simulink model "MassSpringDamper"  (R2015b)
settings: Solver=VariableStepAuto  StartTime=0.0  StopTime=10  RelTol=1e-3
values from neighbouring files (symbols this model uses):
  b = 2    [MassDamperSpring.m]
  F = 1    [MassDamperSpring.m]
  k = 20    [MassDamperSpring.m]
  m = 1    [MassDamperSpring.m]
settings Model: Creator=DCLAP  LastModifiedBy=DCLAP

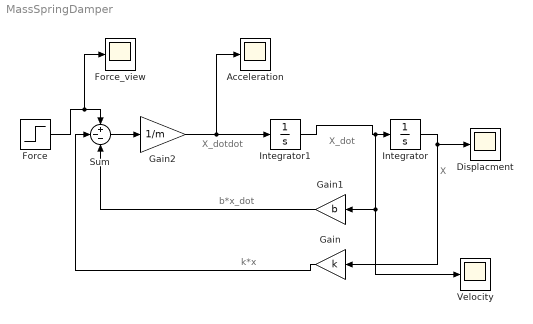
== system MassSpringDamper ==
  note: k*x
  note: b*x_dot
  note: X
  note: X_dot
  note: X_dotdot
  Acceleration : Scope
  Displacment : Scope
  Force : Step  After=F  SampleTime=0
  Force_view : Scope
  Gain : Gain  Gain=k
  Gain1 : Gain  Gain=b
  Gain2 : Gain  Gain=1/m
  Integrator : Integrator
  Integrator1 : Integrator
  Sum : Sum  Inputs=+--
  Velocity : Scope
  wires:
  Gain2/1 -> Acceleration/1, Integrator1/1
  Integrator/1 -> Displacment/1, Gain/1
  Force/1 -> Force_view/1, Sum/1
  Gain1/1 -> Sum/3
  Gain/1 -> Sum/2
  Sum/1 -> Gain2/1
  Integrator1/1 -> Velocity/1, Gain1/1, Integrator/1
